simulink model "main"  (R2021a)
settings: Solver=ode113  StartTime=0.0  StopTime=6*3600  RelTol=1e-13  AbsTol=1e-14
values from neighbouring files (symbols this model uses):
  Const = createSimulinkBus(Const_1)    [initializeData.m]
  Earth = createSimulinkBus(Earth_1)    [initializeData.m]
  Sensors = createSimulinkBus(Sensors_1)    [initializeData.m]
  Spacecraft = createSimulinkBus(Spacecraft_1)    [initializeData.m]
undefined symbols (not defined in the file or in its folder): initCond
libraries: aerolibutil x25, vrlib x22, SADlibrary x22, dspsrcs4 x17, sharedtransform x8, simulink x6, pid_lib x3, simulink_extras x2, sharedTrackingLibrary x2, dspmathops x1, sharedutil x1
(part 1 of 2)
settings Model: SimulationMode=rapid-accelerator  Creator=matteo  LastModifiedBy=matteo
settings SolverCC: ZeroCrossControl=EnableAll  ZeroCrossAlgorithm=Adaptive  AlgebraicLoopSolver=TrustRegion  DecoupledContinuousIntegration=on
settings DebuggingCC: ReadBeforeWriteMsg=DisableAll  WriteAfterWriteMsg=DisableAll  WriteAfterReadMsg=DisableAll  MultiTaskDSMMsg=none  SFMachineParentedDataDiag=warning
settings ModelReferenceCC: UpdateModelReferenceTargets=IfOutOfDate
settings SFSimCC: SFSimEcho=off
settings SimscapeCC: SimscapeNormalizeSystem=off

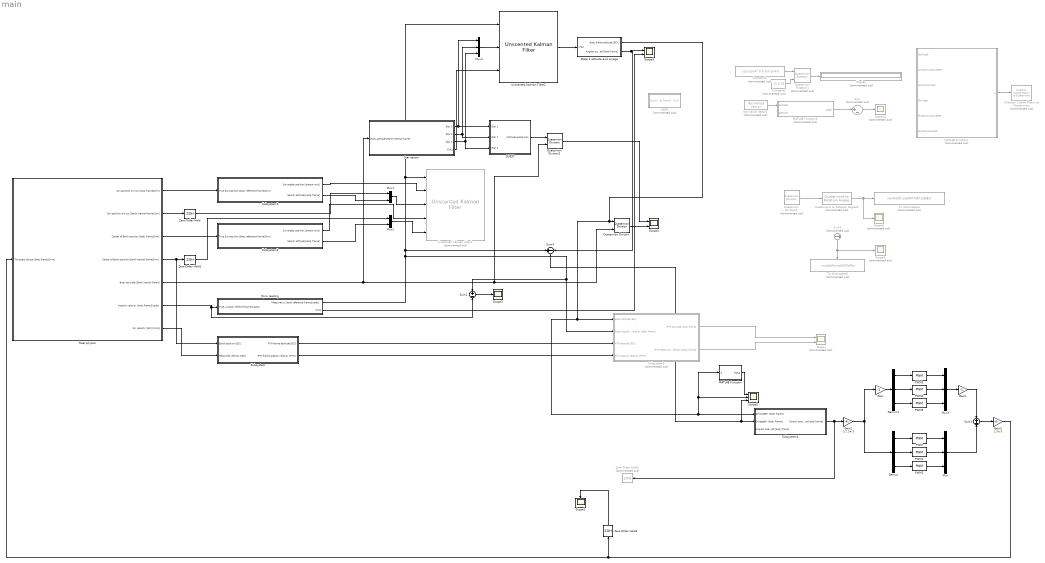
== system main ==
  Constant1 : Constant  Commented=on  Value=[1 0 0]
  Constant3 : Constant  Commented=on  Value=[cos(pi/4) 0 0 sin(pi/4)]
  Demux : Demux  Outputs=3
  Demux1 : Demux  Outputs=3
  Direction Cosine Matrix to Quaternions : sharedtransform/Direction Cosine Matrix  to Quaternions  Commented=on  aMode=0  action=None  tolerance=eps(2)
      settings: SourceProductBaseCode=AE,PW,DR,MT,UV,VE
  Display : Display  Commented=on
  Gain : Gain  Gain=-1
  Gain1 : Gain  Gain=-1
  Gain2 : Gain  Gain=1/2.5e-3
  Gain3 : Gain  Gain=2.5e-3
  Gyro reading : Subsystem
  MATLAB Function : MATLAB Function  TreatAsAtomicUnit=on
  MATLAB Function1 : MATLAB Function  Commented=on  TreatAsAtomicUnit=on
  MATLAB Function3 : MATLAB Function  Commented=on  TreatAsAtomicUnit=on
  MEKF : Subsystem  Commented=on
  Mux : Mux  Inputs=3
  Mux1 : Mux  Inputs=2
  Mux2 : Mux  Inputs=2
  Mux3 : Mux  Inputs=3
  Mux4 : Mux  Inputs=3
  Normalize Vector1 : vrlib/Utilities/Normalize Vector  Commented=on  maxzero=0
  PWM{,1..5} (6 alike) : simulink/Discontinuities/PWM  DisableCoverage=on  Period=.5  DisallowZeroDutyCycle=off  RunAtFixedTimeIntervals=on  SampleTime=.1
  QUEST : Subsystem
  Quaternion Division : aerolibutil/Quaternion Division
      settings: SourceProductBaseCode=AE
  Quaternion Division2 : aerolibutil/Quaternion Division
      settings: SourceProductBaseCode=AE
  Quaternion Division4 : aerolibutil/Quaternion Division  Commented=on
      settings: SourceProductBaseCode=AE
  Quaternion Rotation1 : aerolibutil/Quaternion Rotation  Commented=on
  Quaternions to Rotation Angles3 : sharedtransform/Quaternions to Rotation Angles  Commented=on  rotationOrder=ZYX  aMode=aMode
      settings: SourceProductBaseCode=AE,PW,DR,MT,UV,VE
  Real physics : Subsystem
  Scope : Scope  Commented=on  NumInputPorts=2
  Scope1 : Scope
  Scope10 : Scope  Commented=on
  Scope2 : Scope  NumInputPorts=3
  Scope3 : Scope
  Scope4 : Scope  NumInputPorts=2
  Scope5 : Scope  NumInputPorts=2
  Scope8 : Scope  Commented=on
  Scope9 : Scope  Commented=on
  Star sensor : Subsystem
  State 2 attitude and omega : Subsystem
  Subsystem : Subsystem
  Subsystem1 : Subsystem
  Subsystem2 : Subsystem  Commented=on
  Subsystem3 : Subsystem
  Subsystem4 : Subsystem
  Sum : Sum  Commented=on  Inputs=|+-
  Sum1 : Sum  Inputs=+-
  Sum2 : Sum  Commented=on  Inputs=-+
  Sum3 : Sum
  Sum4 : Sum  Inputs=+-
  To Workspace4 : ToWorkspace  Commented=on  VariableName=nonAdditiveUKFAttitudeErr  SaveFormat=Timeseries  SampleTime=-1
  To Workspace5 : ToWorkspace  Commented=on  VariableName=nonAdditiveUKFVelErr  SaveFormat=Timeseries  SampleTime=-1
  Unscented Kalman Filter1 : sharedTrackingLibrary/Unscented Kalman Filter  Commented=on  StateTransitionFcn=attitudePropagation  HasAdditiveProcessNoise=Nonadditive  ProcessNoise=(1e-1)^2*eye(6)  HasTimeVaryingProcessNoise=off  HasStateTransitionFcnExtraArgument=1  InitialState=[Spacecraft.initialAttitude' 0 0 0]'  InitialStateCovariance=1e-6*eye(7)  Alpha=1e-3  Beta=2  Kappa=0  MeasurementFcn1=simulateSunSensor  HasMeasurementEnablePort1=off  HasAdditiveMeasurementNoise1=Additive  MeasurementNoise1=(.1*pi/180)^2*eye(2)  HasTimeVaryingMeasurementNoise1=off  HasMeasurementFcnExtraArgument1=1  MeasurementFcn2=simulateEarthHorizonSensor  HasMeasurementEnablePort2=off  HasAdditiveMeasurementNoise2=Additive  MeasurementNoise2=(.1*pi/180)^2*eye(2)  HasTimeVaryingMeasurementNoise2=off  HasMeasurementFcnExtraArgument2=1  MeasurementFcn3=simulateSunSensor  HasMeasurementEnablePort3=off  HasAdditiveMeasurementNoise3=Additive  MeasurementNoise3=(.1*pi/180)^2*eye(2)  HasTimeVaryingMeasurementNoise3=off  HasMeasurementFcnExtraArgument3=1  MeasurementFcn4=myMeasurementFcn  HasMeasurementEnablePort4=off  HasAdditiveMeasurementNoise4=Additive  MeasurementNoise4=1  HasTimeVaryingMeasurementNoise4=off  HasMeasurementFcnExtraArgument4=0  MeasurementFcn5=myMeasurementFcn  HasMeasurementEnablePort5=off  HasAdditiveMeasurementNoise5=Additive  MeasurementNoise5=1  HasTimeVaryingMeasurementNoise5=off  HasMeasurementFcnExtraArgument5=0  EnableMultirate=on  StateTransitionFcnSampleTime=.01  MeasurementFcn1SampleTime=Sensors.sunSensorSamplingFreq  MeasurementFcn2SampleTime=Sensors.sunSensorSamplingFreq  MeasurementFcn3SampleTime=Sensors.sunSensorSamplingFreq  MeasurementFcn4SampleTime=1  MeasurementFcn5SampleTime=1  UseCurrentEstimator=on  OutputStateCovariance=off  DataType=double  SampleTime=0.01  NumberOfMeasurements=2
      settings: SourceProductBaseCode=CT,DR,TF,ID,LP,NV,AR,RO,RR,UV,VE
  Unscented Kalman Filter2 : sharedTrackingLibrary/Unscented Kalman Filter  StateTransitionFcn=attitudePropagation  HasAdditiveProcessNoise=Nonadditive  ProcessNoise=(1e-4)^2*eye(6)  HasTimeVaryingProcessNoise=off  HasStateTransitionFcnExtraArgument=1  InitialState=[Spacecraft.initialAttitude' 0 0 0]'  InitialStateCovariance=1e-6*eye(7)  Alpha=1e-3  Beta=2  Kappa=0  MeasurementFcn1=simulateStarSensor  HasMeasurementEnablePort1=off  HasAdditiveMeasurementNoise1=Additive  MeasurementNoise1=(.1*pi/180)^2*eye(6)  HasTimeVaryingMeasurementNoise1=off  HasMeasurementFcnExtraArgument1=1  MeasurementFcn2=simulateEarthHorizonSensor  HasMeasurementEnablePort2=off  HasAdditiveMeasurementNoise2=Additive  MeasurementNoise2=(.1*pi/180)^2*eye(2)  HasTimeVaryingMeasurementNoise2=off  HasMeasurementFcnExtraArgument2=1  MeasurementFcn3=simulateSunSensor  HasMeasurementEnablePort3=off  HasAdditiveMeasurementNoise3=Additive  MeasurementNoise3=(.1*pi/180)^2*eye(2)  HasTimeVaryingMeasurementNoise3=off  HasMeasurementFcnExtraArgument3=1  MeasurementFcn4=myMeasurementFcn  HasMeasurementEnablePort4=off  HasAdditiveMeasurementNoise4=Additive  MeasurementNoise4=1  HasTimeVaryingMeasurementNoise4=off  HasMeasurementFcnExtraArgument4=0  MeasurementFcn5=myMeasurementFcn  HasMeasurementEnablePort5=off  HasAdditiveMeasurementNoise5=Additive  MeasurementNoise5=1  HasTimeVaryingMeasurementNoise5=off  HasMeasurementFcnExtraArgument5=0  EnableMultirate=on  StateTransitionFcnSampleTime=.01  MeasurementFcn1SampleTime=1  MeasurementFcn2SampleTime=Sensors.sunSensorSamplingFreq  MeasurementFcn3SampleTime=Sensors.sunSensorSamplingFreq  MeasurementFcn4SampleTime=1  MeasurementFcn5SampleTime=1  UseCurrentEstimator=off  OutputStateCovariance=off  DataType=double  SampleTime=0.01  NumberOfMeasurements=1
      settings: SourceProductBaseCode=CT,DR,TF,ID,LP,NV,AR,RO,RR,UV,VE
  Zero-Order Hold : ZeroOrderHold  SampleTime=Sensors.sunSensorSamplingFreq
  Zero-Order Hold1 : ZeroOrderHold  SampleTime=Sensors.sunSensorSamplingFreq
  Zero-Order Hold2 : ZeroOrderHold  Commented=on  SampleTime=.01
  Zero-Order Hold3 : ZeroOrderHold  SampleTime=.01
  wires:
  Real physics/6(Angular velocity [body frame][rad/s]) -> Sum1/2, Gyro reading/1(True ω [body refrence frame][rad/s])
  Real physics/2(Sun position wrt s/c [Earth inertial frame][km]) -> Zero-Order Hold/1
  Real physics/4(Center of Earth position [Earth inertial frame][km]) -> Subsystem/1(Earth position [ECI]), Zero-Order Hold1/1
  Sum2/1 -> To Workspace5/1, Scope9/1
  Quaternions to Rotation Angles3/1 -> Scope8/1, To Workspace4/1
  Quaternion Division4/1 -> Quaternions to Rotation Angles3/1
  Real physics/3(Center of Earth position [body frame][km]) -> Subsystem3/1(True Sun position [body reference frame][km])
  Zero-Order Hold/1 -> Mux1/1
  Zero-Order Hold1/1 -> Mux2/1
  Normalize Vector1/1 -> MATLAB Function3/1(earthECI)
  MATLAB Function3/1(angle) -> Sum/1
  Sum/1 -> Scope10/1
  Real physics/7(S/c velocity [ECI][kim/s]) -> Subsystem/2(Measured velocity [ECI])
  Demux/1 -> PWM/1
  Demux/3 -> PWM2/1
  Demux/2 -> PWM1/1
  PWM/1 -> Mux/1
  PWM1/1 -> Mux/2
  PWM2/1 -> Mux/3
  Subsystem1/1(Sun angles position [sensor axis]) -> Unscented Kalman Filter1/2
  Real physics/1(Sun position wrt s/c [body frame][km]) -> Subsystem1/1(True Sun position [body reference frame][km])
  Subsystem3/2(Sensor attitude [body frame]) -> Mux2/2
  Subsystem3/1(Sun angles position [sensor axis]) -> Unscented Kalman Filter1/4
  Subsystem1/2(Sensor attitude [body frame]) -> Mux1/2
  Constant3/1 -> Quaternion Rotation1/1
  Constant1/1 -> Quaternion Rotation1/2
  Quaternion Rotation1/1 -> Display/1
  Mux1/1 -> Unscented Kalman Filter1/3
  Mux2/1 -> Unscented Kalman Filter1/5
  Sum3/1 -> Gain3/1
  State 2 attitude and omega/1(Body frame attitude [ECI]) -> MATLAB Function/1(q), Scope2/2, Subsystem4/1(AttitudeErr [body frame]), Subsystem2/1(Body attitude [ECI]), Quaternion Division/1
  Gyro reading/1(Measured ω [body reference frame][rad/s]) -> Sum4/1, Unscented Kalman Filter2/1, Unscented Kalman Filter1/1, Sum1/1, Subsystem2/2(Body angular velocity [body frame])
  Subsystem/1(RTH frame attitude [ECI]) -> Subsystem2/3(RTH attitude [ECI])
  Subsystem/2("RTH frame angular velocity [RTH] ") -> Subsystem2/4(RTH angular velocity [RTH])
  Subsystem2/1(RTH attitude [body frame]) -> Scope/1
  Subsystem2/2(RTH relative angular velocity [body frame]) -> Scope/2
  Sum1/1 -> Scope3/1
  PWM3/1 -> Mux3/1
  PWM5/1 -> Mux3/3
  Demux1/2 -> PWM4/1
  PWM4/1 -> Mux3/2
  Demux1/1 -> PWM3/1
  Demux1/3 -> PWM5/1
  Gain/1 -> Demux1/1
  Mux3/1 -> Gain1/1
  Gain1/1 -> Sum3/1
  Mux/1 -> Sum3/2
  Subsystem4/1(Control torque [body frame]) -> Zero-Order Hold2/1, Gain2/1
  Zero-Order Hold3/1 -> Scope1/1
  Gain2/1 -> Gain/1, Demux/1
  Gain3/1 -> Zero-Order Hold3/1, Real physics/1(Thrusters torque [body frame][N m])
  MATLAB Function/1(theta) -> Scope2/1
  MATLAB Function1/1(A) -> Direction Cosine Matrix to Quaternions/1
  Real physics/5(Body attitude [Earth inertial frame]) -> Quaternion Division2/2, Quaternion Division/2, Star sensor/1(Body attitude [Earth inertial frame])
  Quaternion Division/1 -> Scope4/2
  Star sensor/1(Star 1) -> Mux4/1, QUEST/1(Star 1)
  Star sensor/2(Star 2) -> QUEST/2(Star 2), Mux4/2
  Star sensor/3(Star 3) -> QUEST/3(Star 3), Mux4/3
  QUEST/1(Attitude quaternion) -> Quaternion Division2/1
  Quaternion Division2/1 -> Scope4/1
  Mux4/1 -> Unscented Kalman Filter2/2
  Star sensor/4(Out1) -> Unscented Kalman Filter2/3
  Unscented Kalman Filter2/1 -> State 2 attitude and omega/1(xHat)
  Gyro reading/2(Out1) -> Scope5/2
  State 2 attitude and omega/2(Angolar speed [body frame]) -> Sum4/2, Scope5/1
  Sum4/1 -> Subsystem4/2(OmegaErr [body frame]), Scope2/3

== system main/Gyro reading ==
  True ω [body refrence frame][rad/s] : Inport
  Cumulative Sum : dspmathops/Cumulative Sum  dim=Channels (running sum)  reset_popup=None  roundingMode=Floor  overflowMode=off  outputDataTypeStr=Inherit: Same as accumulator  outputMin=[]  outputMax=[]  outputLastDataTypeStr=Inherit: Same as accumulator
  Gain : Gain  Gain=sqrt(0.01)
  Random Source : dspsrcs4/Random Source  SrcType=Gaussian  NormMethod=Ziggurat  CltLength=12  MinVal=0  MaxVal=1  MeanVal=0  VarVal=(1e-4)^2  RepMode=Not repeatable  rawSeed=1  IsInherit=off  SampMode=Discrete  SampTime=0.01  SampFrame=3  DataType=Double  OutComplex=Real  OutputFrames=off
  Random Source1 : dspsrcs4/Random Source  SrcType=Gaussian  NormMethod=Ziggurat  CltLength=12  MinVal=0  MaxVal=1  MeanVal=0  VarVal=(1e-4)^2  RepMode=Not repeatable  rawSeed=1  IsInherit=off  SampMode=Discrete  SampTime=0.01  SampFrame=3  DataType=Double  OutComplex=Real  OutputFrames=off
  Sum : Sum  Inputs=+++
  Zero-Order Hold : ZeroOrderHold  SampleTime=.01
  Measured ω [body reference frame][rad/s] : Outport
  Out1 : Outport  Port=2
  wires:
  Sum/1 -> Measured ω [body reference frame][rad/s]/1
  True ω [body refrence frame][rad/s]/1 -> Zero-Order Hold/1
  Zero-Order Hold/1 -> Sum/2
  Cumulative Sum/1 -> Out1/1, Sum/1
  Gain/1 -> Cumulative Sum/1
  Random Source/1 -> Sum/3
  Random Source1/1 -> Gain/1

== system main/MEKF ==
  note: With
      | $G(t)= \left[ \begin{array}{cccccc} -1 \\ & -1 \\ & & -1 \\ & & & 1 \\ & & & & 1 \\ & & & & & 1 \end{array} \right] \quad \text{and} \quad Q(t) = \left[ \begin{array}{cccccc} \sigma_v^2 \\ & \sigma_v^2 \\ & & \sigma_v^2 \\ & & & \sigma_u^2 \\ & & & & \sigma_u^2 \\ & & & & & \sigma_u^2 \end{array} \right]$
  Gyro [rad/s] [body frame] : Inport
  G*Q*G' : Constant  Value="diag([1  1  1  1  1  1 ])"
  Gain : Gain  Gain=0.5
  Integrator : Integrator  InitialConditionSource=external
  Integrator1 : Integrator  InitialConditionSource=external
  MATLAB Function : MATLAB Function  TreatAsAtomicUnit=on
  MATLAB Function1 : MATLAB Function  TreatAsAtomicUnit=on
  MATLAB Function2 : MATLAB Function  TreatAsAtomicUnit=on
  Product : Product
  Product1 : Product
  Product2 : Product
  Sum : Sum  Inputs=+++
  Transpose : Math  Operator=transpose  SaturateOnIntegerOverflow=on
  Out1 : Outport
  wires:
  Gyro [rad/s] [body frame]/1 -> MATLAB Function1/1(v), Out1/1, Product/2
  MATLAB Function/1(Q) -> Product/1
  Product/1 -> Gain/1
  Gain/1 -> Integrator/1
  Integrator/1 -> MATLAB Function/1(q)
  MATLAB Function1/1(vCross) -> MATLAB Function2/1(omegaCross)
  MATLAB Function2/1(F) -> Product1/1, Transpose/1
  Integrator1/1 -> Product1/2, Product2/1
  Transpose/1 -> Product2/2
  Product1/1 -> Sum/2
  Product2/1 -> Sum/3
  Sum/1 -> Integrator1/1
  G*Q*G'/1 -> Sum/1

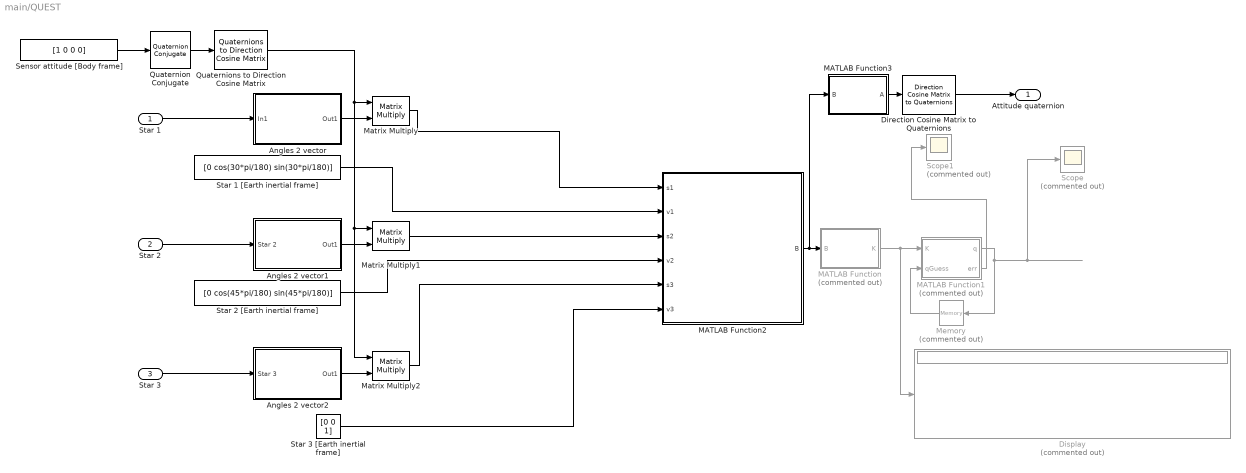
== system main/QUEST ==
  Star 1 : Inport
  Star 2 : Inport  Port=2
  Star 3 : Inport  Port=3
  Angles 2 vector : Subsystem
  Angles 2 vector1 : Subsystem
  Angles 2 vector2 : Subsystem
  Direction Cosine Matrix to Quaternions : sharedtransform/Direction Cosine Matrix  to Quaternions  aMode=0  action=None  tolerance=eps(2)
      settings: SourceProductBaseCode=AE,PW,DR,MT,UV,VE
  Display : Display  Commented=on
  MATLAB Function : MATLAB Function  Commented=on  TreatAsAtomicUnit=on
  MATLAB Function1 : MATLAB Function  Commented=on  TreatAsAtomicUnit=on
  MATLAB Function2 : MATLAB Function  TreatAsAtomicUnit=on
  MATLAB Function3 : MATLAB Function  TreatAsAtomicUnit=on
  Matrix Multiply : Product  Multiplication=Matrix(*)
  Matrix Multiply1 : Product  Multiplication=Matrix(*)
  Matrix Multiply2 : Product  Multiplication=Matrix(*)
  Memory : Memory  Commented=on  InitialCondition=[1 0 0 0]
  Quaternion Conjugate : aerolibutil/Quaternion Conjugate
      settings: SourceProductBaseCode=AE
  Quaternions to Direction Cosine Matrix : sharedtransform/Quaternions to  Direction Cosine Matrix  aMode=aMode
      settings: SourceProductBaseCode=AE,PW,DR,MT,UV,VE
  Scope : Scope  Commented=on
  Scope1 : Scope  Commented=on
  Sensor attitude [Body frame] : Constant  Value=[1 0 0 0]
  Star 1 [Earth inertial frame] : Constant  Value=[0 cos(30*pi/180) sin(30*pi/180)]
  Star 2 [Earth inertial frame] : Constant  Value=[0 cos(45*pi/180) sin(45*pi/180)]
  Star 3 [Earth inertial frame] : Constant  Value=[0 0 1]
  Attitude quaternion : Outport
  wires:
  Star 1/1 -> Angles 2 vector/1(In1)
  Star 2/1 -> Angles 2 vector1/1(Star 2)
  Star 3/1 -> Angles 2 vector2/1(Star 3)
  Star 1 [Earth inertial frame]/1 -> MATLAB Function2/2(v1)
  Angles 2 vector/1(Out1) -> Matrix Multiply/2
  Star 2 [Earth inertial frame]/1 -> MATLAB Function2/4(v2)
  Star 3 [Earth inertial frame]/1 -> MATLAB Function2/6(v3)
  MATLAB Function2/1(B) -> MATLAB Function3/1(B), MATLAB Function/1(B)
  MATLAB Function/1(K) -> Display/1, MATLAB Function1/1(K)
  MATLAB Function1/1(q) -> Memory/1, Scope/1
  Sensor attitude [Body frame]/1 -> Quaternion Conjugate/1
  Quaternion Conjugate/1 -> Quaternions to Direction Cosine Matrix/1
  Quaternions to Direction Cosine Matrix/1 -> Matrix Multiply2/1, Matrix Multiply1/1, Matrix Multiply/1
  Matrix Multiply/1 -> MATLAB Function2/1(s1)
  Angles 2 vector2/1(Out1) -> Matrix Multiply2/2
  Matrix Multiply2/1 -> MATLAB Function2/5(s3)
  Matrix Multiply1/1 -> MATLAB Function2/3(s2)
  Angles 2 vector1/1(Out1) -> Matrix Multiply1/2
  Memory/1 -> MATLAB Function1/2(qGuess)
  MATLAB Function1/2(err) -> Scope1/1
  MATLAB Function3/1(A) -> Direction Cosine Matrix to Quaternions/1
  Direction Cosine Matrix to Quaternions/1 -> Attitude quaternion/1

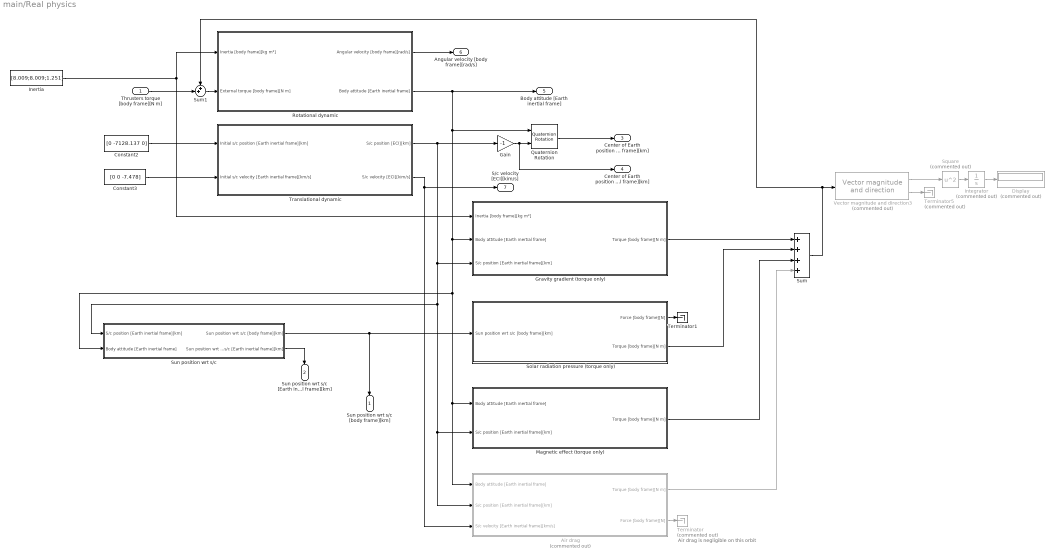
== system main/Real physics ==
  note: Air drag is negligible on this orbit
  Thrusters torque [body frame][N m] : Inport  Unit=N*m
  Air drag : Subsystem  Commented=on
  Constant2 : Constant  Value=[0 -7128.137 0]
  Constant3 : Constant  Value=[0 0 -7.478]
  Display : Display  Commented=on
  Gain : Gain  Gain=-1
  Gravity gradient (torque only) : Subsystem
      settings: PortSchema="{\"entries\":[{\"content\":{\"sides\":[{\"content\":{\"connectorIds\":[\"Out1\"]},\"type\":\"ConnectorPlacement.EquallySpacedRectSide\",\"uuid\":\"f1f9fb06-69b8-4265-b1e3-1bc99765f445\"},{\"content\":{\"connectorIds\":[\"In1\",\"In2\",\"In3\"],\"side\":\"RIGHT\"},\"type\":\"ConnectorPlacement.EquallySpacedRectSide\",\"uuid\":\"95872401-8fe8-493a-a743-72ee2e043305\"},{\"content\":{\"connectorIds\":[],\"side\":\"TOP\"},\"type\":\"ConnectorPlacement.EquallySpacedRectSide\",\"uuid\":\"a2f933f3-d116-4556-b216-8e543aff18f5\"},{\"content\":{\"connectorIds\":[],\"side\":\"HIDDEN\"},\"type\":\"ConnectorPlacement.EquallySpacedRectSide\",\"uuid\":\"93d45030-e624-494e-a335-b0ea445a7c18\"}]},\"type\":\"ConnectorPlacement.EquallySpacedConnector\",\"uuid\":\"bbb7bc93-29be-48e8-9ed7-f6b41cc2b7e1\"}],\"packageUris\":[\"http://schema.mathworks.com/mf0/Connector/R2020b\"],\"version\":\"1.0\"}"
  Inertia : Constant  Value=[8.009;8.009;1.251]
  Integrator : Integrator  Commented=on
  Magnetic effect (torque only) : Subsystem
  Quaternion Rotation : aerolibutil/Quaternion Rotation
  Rotational dynamic : Subsystem
  Solar radiation pressure (torque only) : Subsystem
  Square : Math  Commented=on  Operator=square  SaturateOnIntegerOverflow=on
  Sum : Sum  Inputs=++++
  Sum1 : Sum  Inputs=++|
  Sun position wrt s/c : Subsystem
  Terminator : Terminator  Commented=on
  Terminator1 : Terminator
  Terminator5 : Terminator  Commented=on
  Translational dynamic : Subsystem
  Vector magnitude and direction3 : SADlibrary/Vector magnitude and direction  Commented=on  SystemSampleTime=-1  VariantActivationTime=update diagram  Latency=0  AutoFrameSizeCalculation=off
  Sun position wrt s/c [body frame][km] : Outport  OutDataTypeStr=double  Unit=km
  Sun position wrt s/c [Earth inertial frame][km] : Outport  Port=2
  Center of Earth position [body frame][km] : Outport  Port=3
  Center of Earth position [Earth inertial frame][km] : Outport  Port=4
  Body attitude [Earth inertial frame] : Outport  Port=5
  Angular velocity [body frame][rad/s] : Outport  Port=6
  S/c velocity [ECI][kim/s] : Outport  Port=7
  wires:
  Inertia/1 -> Gravity gradient (torque only)/1(Inertia [body frame][kg m²]), Rotational dynamic/1(Inertia [body frame][kg m²])
  Rotational dynamic/1(Angular velocity [body frame][rad/s]) -> Angular velocity [body frame][rad/s]/1
  Constant2/1 -> Translational dynamic/1(Initial s/c position [Earth inertial frame][km])
  Constant3/1 -> Translational dynamic/2(Initial s/c velocity [Earth inertial frame][km/s])
  Rotational dynamic/2(Body attitude [Earth inertial frame]) -> Body attitude [Earth inertial frame]/1, Quaternion Rotation/1, Air drag/1(Body attitude [Earth inertial frame]), Magnetic effect (torque only)/1(Body attitude [Earth inertial frame]), Sun position wrt s/c/2(Body attitude [Earth inertial frame]), Gravity gradient (torque only)/2(Body attitude [Earth inertial frame])
  Translational dynamic/1(S/c position [ECI][km]) -> Gain/1, Gravity gradient (torque only)/3(S/c position [Earth inertial frame][km]), Sun position wrt s/c/1(S/c position [Earth inertial frame][km]), Air drag/2(S/c position [Earth inertial frame][km]), Magnetic effect (torque only)/2(S/c position [Earth inertial frame][km])
  Sum/1 -> Sum1/1, Vector magnitude and direction3/1
  Air drag/2(Force [body frame][N]) -> Terminator/1
  Solar radiation pressure (torque only)/1(Force [body frame][N]) -> Terminator1/1
  Sun position wrt s/c/1(Sun position wrt s/c [body frame][km]) -> Solar radiation pressure (torque only)/1(Sun position wrt s/c [body frame][km]), Sun position wrt s/c [body frame][km]/1
  Solar radiation pressure (torque only)/2(Torque [body frame][N m]) -> Sum/2
  Magnetic effect (torque only)/1(Torque [body frame][N m]) -> Sum/3
  Air drag/1(Torque [body frame][N m]) -> Sum/4
  Gravity gradient (torque only)/1(Torque [body frame][N m]) -> Sum/1
  Gain/1 -> Center of Earth position [Earth inertial frame][km]/1, Quaternion Rotation/2
  Quaternion Rotation/1 -> Center of Earth position [body frame][km]/1
  Sun position wrt s/c/2(Sun position wrt s/c [Earth inertial frame][km]) -> Sun position wrt s/c [Earth inertial frame][km]/1
  Thrusters torque [body frame][N m]/1 -> Sum1/2
  Sum1/1 -> Rotational dynamic/2(External torque [body frame][N m])
  Vector magnitude and direction3/1 -> Square/1
  Vector magnitude and direction3/2 -> Terminator5/1
  Square/1 -> Integrator/1
  Integrator/1 -> Display/1
  Translational dynamic/2(S/c velocity [ECI][kim/s]) -> S/c velocity [ECI][kim/s]/1, Air drag/3(S/c velocity [Earth inertial frame][km/s])

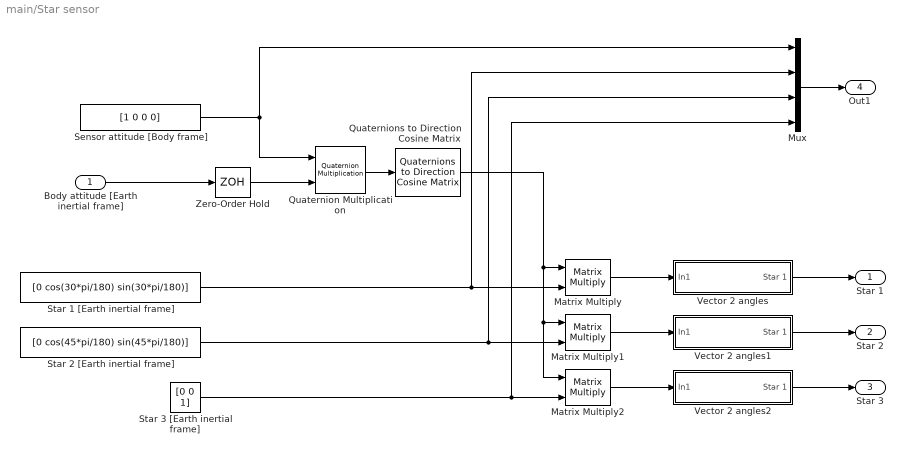
== system main/Star sensor ==
  Body attitude [Earth inertial frame] : Inport
  Matrix Multiply : Product  Multiplication=Matrix(*)
  Matrix Multiply1 : Product  Multiplication=Matrix(*)
  Matrix Multiply2 : Product  Multiplication=Matrix(*)
  Mux : Mux
  Quaternion Multiplication : aerolibutil/Quaternion Multiplication
  Quaternions to Direction Cosine Matrix : sharedtransform/Quaternions to  Direction Cosine Matrix  aMode=aMode
      settings: SourceProductBaseCode=AE,PW,DR,MT,UV,VE
  Sensor attitude [Body frame] : Constant  Value=[1 0 0 0]
  Star 1 [Earth inertial frame] : Constant  Value=[0 cos(30*pi/180) sin(30*pi/180)]
  Star 2 [Earth inertial frame] : Constant  Value=[0 cos(45*pi/180) sin(45*pi/180)]
  Star 3 [Earth inertial frame] : Constant  Value=[0 0 1]
  Vector 2 angles : Subsystem
  Vector 2 angles1 : Subsystem
  Vector 2 angles2 : Subsystem
  Zero-Order Hold : ZeroOrderHold
  Star 1 : Outport
  Star 2 : Outport  Port=2
  Star 3 : Outport  Port=3
  Out1 : Outport  Port=4
  wires:
  Body attitude [Earth inertial frame]/1 -> Zero-Order Hold/1
  Sensor attitude [Body frame]/1 -> Mux/1, Quaternion Multiplication/1
  Quaternion Multiplication/1 -> Quaternions to Direction Cosine Matrix/1
  Star 1 [Earth inertial frame]/1 -> Matrix Multiply/2, Mux/2
  Star 2 [Earth inertial frame]/1 -> Mux/3, Matrix Multiply1/2
  Star 3 [Earth inertial frame]/1 -> Mux/4, Matrix Multiply2/2
  Quaternions to Direction Cosine Matrix/1 -> Matrix Multiply2/1, Matrix Multiply1/1, Matrix Multiply/1
  Matrix Multiply/1 -> Vector 2 angles/1(In1)
  Matrix Multiply2/1 -> Vector 2 angles2/1(In1)
  Matrix Multiply1/1 -> Vector 2 angles1/1(In1)
  Vector 2 angles1/1(Star 1) -> Star 2/1
  Vector 2 angles2/1(Star 1) -> Star 3/1
  Vector 2 angles/1(Star 1) -> Star 1/1
  Mux/1 -> Out1/1
  Zero-Order Hold/1 -> Quaternion Multiplication/2

== system main/State 2 attitude and omega ==
  xHat : Inport
  Demux1 : Demux  Outputs=7
  Mux2 : Mux
  Mux3 : Mux  Inputs=3
  Body frame attitude [ECI] : Outport
  Angolar speed [body frame] : Outport  Port=2
  wires:
  Mux2/1 -> Body frame attitude [ECI]/1
  Demux1/2 -> Mux2/2
  Mux3/1 -> Angolar speed [body frame]/1
  Demux1/7 -> Mux3/3
  Demux1/1 -> Mux2/1
  Demux1/3 -> Mux2/3
  Demux1/5 -> Mux3/1
  xHat/1 -> Demux1/1
  Demux1/6 -> Mux3/2
  Demux1/4 -> Mux2/4

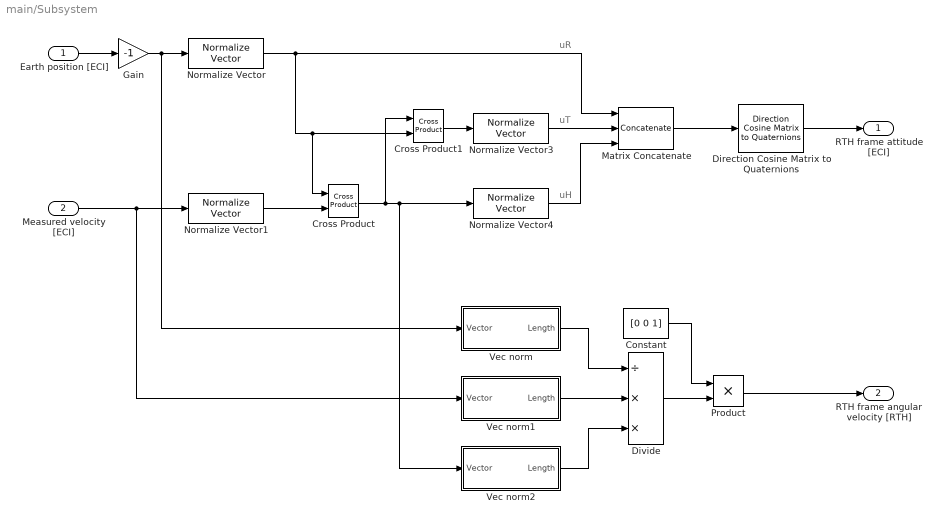
== system main/Subsystem ==
  note: uR
  note: uT
  note: uH
  Earth position [ECI] : Inport
  Measured velocity [ECI] : Inport  Port=2
  Constant : Constant  Value=[0 0 1]
  Cross Product : vrlib/Utilities/Cross Product
  Cross Product1 : vrlib/Utilities/Cross Product
  Direction Cosine Matrix to Quaternions : sharedtransform/Direction Cosine Matrix  to Quaternions  aMode=0  action=None  tolerance=eps(2)
      settings: SourceProductBaseCode=AE,PW,DR,MT,UV,VE
  Divide : Product  Inputs=/**
  Gain : Gain  Gain=-1
  Matrix Concatenate : Concatenate  NumInputs=3  Mode=Multidimensional array  ConcatenateDimension=2
  Normalize Vector{,1,3..4} (4 alike) : vrlib/Utilities/Normalize Vector  maxzero=0
  Product : Product
  Vec norm : Subsystem
  Vec norm1 : Subsystem
  Vec norm2 : Subsystem
  RTH frame attitude [ECI] : Outport
  "RTH frame angular velocity [RTH] " : Outport  Port=2
  wires:
  Matrix Concatenate/1 -> Direction Cosine Matrix to Quaternions/1
  Direction Cosine Matrix to Quaternions/1 -> RTH frame attitude [ECI]/1
  Earth position [ECI]/1 -> Gain/1
  Cross Product/1 -> Vec norm2/1(Vector), Normalize Vector4/1, Cross Product1/1
  Normalize Vector/1 -> Matrix Concatenate/1, Cross Product/1, Cross Product1/2
  Normalize Vector4/1 -> Matrix Concatenate/3
  Normalize Vector3/1 -> Matrix Concatenate/2
  Measured velocity [ECI]/1 -> Vec norm1/1(Vector), Normalize Vector1/1
  Cross Product1/1 -> Normalize Vector3/1
  Vec norm/1(Length) -> Divide/1
  Vec norm1/1(Length) -> Divide/2
  Vec norm2/1(Length) -> Divide/3
  Divide/1 -> Product/2
  Product/1 -> "RTH frame angular velocity [RTH] "/1
  Normalize Vector1/1 -> Cross Product/2
  Gain/1 -> Normalize Vector/1, Vec norm/1(Vector)
  Constant/1 -> Product/1

== system main/Subsystem1 ==
  True Sun position [body reference frame][km] : Inport
  MATLAB Function1 : MATLAB Function  TreatAsAtomicUnit=on
  Sun sensor reading1 : Subsystem
  Sun sensor reading2 : Subsystem
  Sun sensor reading3 : Subsystem
  Sun sensor reading4 : Subsystem
  Sun sensor reading5 : Subsystem
  Sun sensor reading6 : Subsystem
  Sun angles position [sensor axis] : Outport  PortDimensions=2
  Sensor attitude [body frame] : Outport  Port=2  PortDimensions=4
  wires:
  True Sun position [body reference frame][km]/1 -> Sun sensor reading3/1(True Sun position [body reference frame][km]), Sun sensor reading1/1(True Sun position [body reference frame][km]), Sun sensor reading2/1(True Sun position [body reference frame][km]), Sun sensor reading6/1(True Sun position [body reference frame][km]), Sun sensor reading5/1(True Sun position [body reference frame][km]), Sun sensor reading4/1(True Sun position [body reference frame][km])
  MATLAB Function1/2(sensAtt) -> Sensor attitude [body frame]/1
  Sun sensor reading2/1(Sun angles position [sensor axis]) -> MATLAB Function1/2(s2)
  Sun sensor reading1/1(Sun angles position [sensor axis]) -> MATLAB Function1/1(s1)
  Sun sensor reading3/1(Sun angles position [sensor axis]) -> MATLAB Function1/3(s3)
  Sun sensor reading4/1(Sun angles position [sensor axis]) -> MATLAB Function1/4(s4)
  Sun sensor reading5/1(Sun angles position [sensor axis]) -> MATLAB Function1/5(s5)
  Sun sensor reading6/1(Sun angles position [sensor axis]) -> MATLAB Function1/6(s6)
  MATLAB Function1/1(s) -> Sun angles position [sensor axis]/1

== system main/Subsystem2 ==
  Body attitude [ECI] : Inport
  Body angular velocity [body frame] : Inport  Port=2
  RTH attitude [ECI] : Inport  Port=3
  RTH angular velocity [RTH] : Inport  Port=4
  Quaternion Conjugate : aerolibutil/Quaternion Conjugate
      settings: SourceProductBaseCode=AE
  Quaternion Multiplication : aerolibutil/Quaternion Multiplication
  Quaternion Rotation : aerolibutil/Quaternion Rotation
  Sum1 : Sum  Inputs=+-
  RTH attitude [body frame] : Outport
  RTH relative angular velocity [body frame] : Outport  Port=2
  wires:
  Sum1/1 -> RTH relative angular velocity [body frame]/1
  Body angular velocity [body frame]/1 -> Sum1/2
  RTH attitude [ECI]/1 -> Quaternion Multiplication/1
  RTH angular velocity [RTH]/1 -> Quaternion Rotation/2
  Body attitude [ECI]/1 -> Quaternion Conjugate/1
  Quaternion Rotation/1 -> Sum1/1
  Quaternion Multiplication/1 -> Quaternion Rotation/1, RTH attitude [body frame]/1
  Quaternion Conjugate/1 -> Quaternion Multiplication/2

== system main/Subsystem3 ==
  True Sun position [body reference frame][km] : Inport
  MATLAB Function1 : MATLAB Function  TreatAsAtomicUnit=on
  Sun sensor reading1 : Subsystem
  Sun sensor reading2 : Subsystem
  Sun sensor reading3 : Subsystem
  Sun sensor reading4 : Subsystem
  Sun sensor reading5 : Subsystem
  Sun sensor reading6 : Subsystem
  Sun angles position [sensor axis] : Outport  PortDimensions=2
  Sensor attitude [body frame] : Outport  Port=2  PortDimensions=4
  wires:
  True Sun position [body reference frame][km]/1 -> Sun sensor reading3/1(True Sun position [body reference frame][km]), Sun sensor reading1/1(True Sun position [body reference frame][km]), Sun sensor reading2/1(True Sun position [body reference frame][km]), Sun sensor reading6/1(True Sun position [body reference frame][km]), Sun sensor reading5/1(True Sun position [body reference frame][km]), Sun sensor reading4/1(True Sun position [body reference frame][km])
  MATLAB Function1/2(sensAtt) -> Sensor attitude [body frame]/1
  Sun sensor reading2/1(Sun angles position [sensor axis]) -> MATLAB Function1/2(s2)
  Sun sensor reading1/1(Sun angles position [sensor axis]) -> MATLAB Function1/1(s1)
  Sun sensor reading3/1(Sun angles position [sensor axis]) -> MATLAB Function1/3(s3)
  Sun sensor reading4/1(Sun angles position [sensor axis]) -> MATLAB Function1/4(s4)
  Sun sensor reading5/1(Sun angles position [sensor axis]) -> MATLAB Function1/5(s5)
  Sun sensor reading6/1(Sun angles position [sensor axis]) -> MATLAB Function1/6(s6)
  MATLAB Function1/1(s) -> Sun angles position [sensor axis]/1

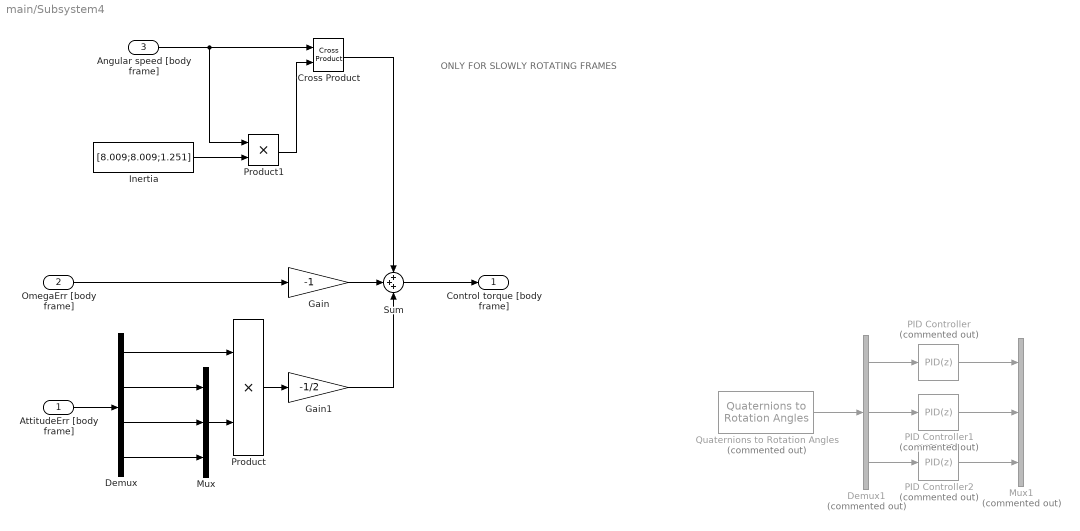
== system main/Subsystem4 ==
  note: ONLY FOR SLOWLY ROTATING FRAMES
  AttitudeErr [body frame] : Inport
  OmegaErr [body frame] : Inport  Port=2
  Angular speed [body frame] : Inport  Port=3
  Cross Product : vrlib/Utilities/Cross Product
  Demux : Demux
  Demux1 : Demux  Commented=on  Outputs=3
  Gain : Gain  Gain=-1
  Gain1 : Gain  Gain=-1/2
  Inertia : Constant  Value=[8.009;8.009;1.251]
  Mux : Mux  Inputs=3
  Mux1 : Mux  Commented=on  Inputs=3
  PID Controller : pid_lib/PID Controller  Commented=on  Controller=PID  Form=Parallel  TimeDomain=Discrete-time  UseExternalTs=off  SampleTime=-1  IntegratorMethod=Forward Euler  FilterMethod=Forward Euler  ControllerParametersSource=internal  P=1  I=1  D=0  UseFilter=on  N=100  TunerSelectOption=Transfer Function Based (PID Tuner App)  InitialConditionSource=internal  InitialConditionForIntegrator=0  InitialConditionForFilter=0  DifferentiatorICPrevScaledInput=0  ExternalReset=none  TrackingMode=off  Kt=1  LimitOutput=off  SatLimitsSource=internal  UpperSaturationLimit=inf  LowerSaturationLimit=-inf  LinearizeAsGain=on  AntiWindupMode=none  Kb=1  POutMin=[]  POutMax=[]  IOutMin=[]  IOutMax=[]  DOutMin=[]  DOutMax=[]  NOutMin=[]  NOutMax=[]  SumOutMin=[]  SumOutMax=[]  SaturationOutMin=[]  SaturationOutMax=[]  PParamMin=[]  PParamMax=[]  IParamMin=[]  IParamMax=[]  DParamMin=[]  DParamMax=[]  NParamMin=[]  NParamMax=[]  KbParamMin=[]  KbParamMax=[]  KtParamMin=[]  KtParamMax=[]  KbOutMin=[]  KbOutMax=[]  KtOutMin=[]  KtOutMax=[]  IntegratorOutMin=[]  IntegratorOutMax=[]  FilterOutMin=[]  FilterOutMax=[]  SumI1OutMin=[]  SumI1OutMax=[]  SumI2OutMin=[]  SumI2OutMax=[]  SumI3OutMin=[]  SumI3OutMax=[]  SumI4OutMin=[]  SumI4OutMax=[]  SumDOutMin=[]  SumDOutMax=[]  DifferentiatorOutMin=[]  DifferentiatorOutMax=[]  FilterDiffOutCoefMin=[]  FilterDiffOutCoefMax=[]  ReciprocalOutMin=[]  ReciprocalOutMax=[]  SumDenOutMin=[]  SumDenOutMax=[]  SumNumOutMin=[]  SumNumOutMax=[]  DivideOutMin=[]  DivideOutMax=[]  UdiffTsProdOutMin=[]  UdiffTsProdOutMax=[]  NTsProdOutMin=[]  NTsProdOutMax=[]  UintegralTsProdOutMin=[]  UintegralTsProdOutMax=[]  UngainTsProdOutMin=[]  UngainTsProdOutMax=[]  IntegratorContinuousStateAttributes=''  IntegratorStateMustResolveToSignalObject=off  IntegratorRTWStateStorageClass=Auto  FilterContinuousStateAttributes=''  FilterStateMustResolveToSignalObject=off  FilterRTWStateStorageClass=Auto  ParallelPVariant=InternalParameters  IdealPVariant=Disabled  IVariant=InternalParameters  DVariant=InternalParameters  IntegratorVariant=Discrete  SatVariant=Disabled  AWVariant=Passthrough  PCopyVariant=Disabled  TRVariant=Disabled  FdbkBlocksVariant=Forward  IdealPFdbkVariant=Disabled  SatFdbkVariant=Disabled  DerivativeFilterVariant=ForwardEulerFilter  NVariant=InternalParameters  NCopyVariant=Disabled  FilterICVariant=InternalICsFilter  IntegratorICVariant=InternalICs  ExternalResetVariant=Disabled  TRSumVariant=Passthrough  SumFdbkVariant=Disabled  SumVariant=Sum_PID  TsampFilterVariant=InternalTs  TsampNgainVariant=Passthrough  TsampIntegralVariant=Passthrough  ExternalSaturationOutDataTypeStr=Inherit: Same as second input
  PID Controller1 : pid_lib/PID Controller  Commented=on  Controller=PID  Form=Parallel  TimeDomain=Discrete-time  UseExternalTs=off  SampleTime=-1  IntegratorMethod=Forward Euler  FilterMethod=Forward Euler  ControllerParametersSource=internal  P=1  I=1  D=0  UseFilter=on  N=100  TunerSelectOption=Transfer Function Based (PID Tuner App)  InitialConditionSource=internal  InitialConditionForIntegrator=0  InitialConditionForFilter=0  DifferentiatorICPrevScaledInput=0  ExternalReset=none  TrackingMode=off  Kt=1  LimitOutput=off  SatLimitsSource=internal  UpperSaturationLimit=inf  LowerSaturationLimit=-inf  LinearizeAsGain=on  AntiWindupMode=none  Kb=1  POutMin=[]  POutMax=[]  IOutMin=[]  IOutMax=[]  DOutMin=[]  DOutMax=[]  NOutMin=[]  NOutMax=[]  SumOutMin=[]  SumOutMax=[]  SaturationOutMin=[]  SaturationOutMax=[]  PParamMin=[]  PParamMax=[]  IParamMin=[]  IParamMax=[]  DParamMin=[]  DParamMax=[]  NParamMin=[]  NParamMax=[]  KbParamMin=[]  KbParamMax=[]  KtParamMin=[]  KtParamMax=[]  KbOutMin=[]  KbOutMax=[]  KtOutMin=[]  KtOutMax=[]  IntegratorOutMin=[]  IntegratorOutMax=[]  FilterOutMin=[]  FilterOutMax=[]  SumI1OutMin=[]  SumI1OutMax=[]  SumI2OutMin=[]  SumI2OutMax=[]  SumI3OutMin=[]  SumI3OutMax=[]  SumI4OutMin=[]  SumI4OutMax=[]  SumDOutMin=[]  SumDOutMax=[]  DifferentiatorOutMin=[]  DifferentiatorOutMax=[]  FilterDiffOutCoefMin=[]  FilterDiffOutCoefMax=[]  ReciprocalOutMin=[]  ReciprocalOutMax=[]  SumDenOutMin=[]  SumDenOutMax=[]  SumNumOutMin=[]  SumNumOutMax=[]  DivideOutMin=[]  DivideOutMax=[]  UdiffTsProdOutMin=[]  UdiffTsProdOutMax=[]  NTsProdOutMin=[]  NTsProdOutMax=[]  UintegralTsProdOutMin=[]  UintegralTsProdOutMax=[]  UngainTsProdOutMin=[]  UngainTsProdOutMax=[]  IntegratorContinuousStateAttributes=''  IntegratorStateMustResolveToSignalObject=off  IntegratorRTWStateStorageClass=Auto  FilterContinuousStateAttributes=''  FilterStateMustResolveToSignalObject=off  FilterRTWStateStorageClass=Auto  ParallelPVariant=InternalParameters  IdealPVariant=Disabled  IVariant=InternalParameters  DVariant=InternalParameters  IntegratorVariant=Discrete  SatVariant=Disabled  AWVariant=Passthrough  PCopyVariant=Disabled  TRVariant=Disabled  FdbkBlocksVariant=Forward  IdealPFdbkVariant=Disabled  SatFdbkVariant=Disabled  DerivativeFilterVariant=ForwardEulerFilter  NVariant=InternalParameters  NCopyVariant=Disabled  FilterICVariant=InternalICsFilter  IntegratorICVariant=InternalICs  ExternalResetVariant=Disabled  TRSumVariant=Passthrough  SumFdbkVariant=Disabled  SumVariant=Sum_PID  TsampFilterVariant=InternalTs  TsampNgainVariant=Passthrough  TsampIntegralVariant=Passthrough  ExternalSaturationOutDataTypeStr=Inherit: Same as second input
  PID Controller2 : pid_lib/PID Controller  Commented=on  Controller=PID  Form=Parallel  TimeDomain=Discrete-time  UseExternalTs=off  SampleTime=-1  IntegratorMethod=Forward Euler  FilterMethod=Forward Euler  ControllerParametersSource=internal  P=1  I=1  D=0  UseFilter=on  N=100  TunerSelectOption=Transfer Function Based (PID Tuner App)  InitialConditionSource=internal  InitialConditionForIntegrator=0  InitialConditionForFilter=0  DifferentiatorICPrevScaledInput=0  ExternalReset=none  TrackingMode=off  Kt=1  LimitOutput=off  SatLimitsSource=internal  UpperSaturationLimit=inf  LowerSaturationLimit=-inf  LinearizeAsGain=on  AntiWindupMode=none  Kb=1  POutMin=[]  POutMax=[]  IOutMin=[]  IOutMax=[]  DOutMin=[]  DOutMax=[]  NOutMin=[]  NOutMax=[]  SumOutMin=[]  SumOutMax=[]  SaturationOutMin=[]  SaturationOutMax=[]  PParamMin=[]  PParamMax=[]  IParamMin=[]  IParamMax=[]  DParamMin=[]  DParamMax=[]  NParamMin=[]  NParamMax=[]  KbParamMin=[]  KbParamMax=[]  KtParamMin=[]  KtParamMax=[]  KbOutMin=[]  KbOutMax=[]  KtOutMin=[]  KtOutMax=[]  IntegratorOutMin=[]  IntegratorOutMax=[]  FilterOutMin=[]  FilterOutMax=[]  SumI1OutMin=[]  SumI1OutMax=[]  SumI2OutMin=[]  SumI2OutMax=[]  SumI3OutMin=[]  SumI3OutMax=[]  SumI4OutMin=[]  SumI4OutMax=[]  SumDOutMin=[]  SumDOutMax=[]  DifferentiatorOutMin=[]  DifferentiatorOutMax=[]  FilterDiffOutCoefMin=[]  FilterDiffOutCoefMax=[]  ReciprocalOutMin=[]  ReciprocalOutMax=[]  SumDenOutMin=[]  SumDenOutMax=[]  SumNumOutMin=[]  SumNumOutMax=[]  DivideOutMin=[]  DivideOutMax=[]  UdiffTsProdOutMin=[]  UdiffTsProdOutMax=[]  NTsProdOutMin=[]  NTsProdOutMax=[]  UintegralTsProdOutMin=[]  UintegralTsProdOutMax=[]  UngainTsProdOutMin=[]  UngainTsProdOutMax=[]  IntegratorContinuousStateAttributes=''  IntegratorStateMustResolveToSignalObject=off  IntegratorRTWStateStorageClass=Auto  FilterContinuousStateAttributes=''  FilterStateMustResolveToSignalObject=off  FilterRTWStateStorageClass=Auto  ParallelPVariant=InternalParameters  IdealPVariant=Disabled  IVariant=InternalParameters  DVariant=InternalParameters  IntegratorVariant=Discrete  SatVariant=Disabled  AWVariant=Passthrough  PCopyVariant=Disabled  TRVariant=Disabled  FdbkBlocksVariant=Forward  IdealPFdbkVariant=Disabled  SatFdbkVariant=Disabled  DerivativeFilterVariant=ForwardEulerFilter  NVariant=InternalParameters  NCopyVariant=Disabled  FilterICVariant=InternalICsFilter  IntegratorICVariant=InternalICs  ExternalResetVariant=Disabled  TRSumVariant=Passthrough  SumFdbkVariant=Disabled  SumVariant=Sum_PID  TsampFilterVariant=InternalTs  TsampNgainVariant=Passthrough  TsampIntegralVariant=Passthrough  ExternalSaturationOutDataTypeStr=Inherit: Same as second input
  Product : Product
  Product1 : Product
  Quaternions to Rotation Angles : sharedtransform/Quaternions to Rotation Angles  Commented=on  rotationOrder=XYZ  aMode=aMode
      settings: SourceProductBaseCode=AE,PW,DR,MT,UV,VE
  Sum : Sum  Inputs=+++
  Control torque [body frame] : Outport
  wires:
  Mux/1 -> Product/2
  Demux/1 -> Product/1
  Quaternions to Rotation Angles/1 -> Demux1/1
  Demux1/1 -> PID Controller/1
  Demux1/2 -> PID Controller1/1
  Demux1/3 -> PID Controller2/1
  PID Controller/1 -> Mux1/1
  PID Controller1/1 -> Mux1/2
  PID Controller2/1 -> Mux1/3
  OmegaErr [body frame]/1 -> Gain/1
  Sum/1 -> Control torque [body frame]/1
  AttitudeErr [body frame]/1 -> Demux/1
  Demux/2 -> Mux/1
  Demux/3 -> Mux/2
  Demux/4 -> Mux/3
  Product/1 -> Gain1/1
  Angular speed [body frame]/1 -> Product1/1, Cross Product/1
  Inertia/1 -> Product1/2
  Product1/1 -> Cross Product/2
  Cross Product/1 -> Sum/1
  Gain/1 -> Sum/2
  Gain1/1 -> Sum/3

== system main/QUEST/Angles 2 vector ==
  In1 : Inport
  Constant : Constant
  Demux : Demux  Outputs=2
  Demux1 : Demux  Outputs=3
  Divide : Product  Inputs=/*
  Mux : Mux  Inputs=3
  Sqrt : Sqrt  SaturateOnIntegerOverflow=on
  Square : Math  Operator=square  SaturateOnIntegerOverflow=on
  Sum : Sum  Inputs=+++
  Tan : Trigonometry  Operator=tan
  Out1 : Outport
  wires:
  Divide/1 -> Out1/1
  Square/1 -> Demux1/1
  Demux1/3 -> Sum/3
  Sum/1 -> Sqrt/1
  Demux/2 -> Mux/2
  Mux/1 -> Divide/2, Square/1
  Demux1/2 -> Sum/2
  In1/1 -> Tan/1
  Demux/1 -> Mux/1
  Sqrt/1 -> Divide/1
  Constant/1 -> Mux/3
  Tan/1 -> Demux/1
  Demux1/1 -> Sum/1

== system main/QUEST/Angles 2 vector1 ==
  Star 2 : Inport
  Constant : Constant
  Demux : Demux  Outputs=2
  Demux1 : Demux  Outputs=3
  Divide : Product  Inputs=/*
  Mux : Mux  Inputs=3
  Sqrt : Sqrt  SaturateOnIntegerOverflow=on
  Square : Math  Operator=square  SaturateOnIntegerOverflow=on
  Sum : Sum  Inputs=+++
  Tan : Trigonometry  Operator=tan
  Out1 : Outport
  wires:
  Divide/1 -> Out1/1
  Square/1 -> Demux1/1
  Demux1/3 -> Sum/3
  Sum/1 -> Sqrt/1
  Demux/2 -> Mux/2
  Mux/1 -> Divide/2, Square/1
  Demux1/2 -> Sum/2
  Star 2/1 -> Tan/1
  Demux/1 -> Mux/1
  Sqrt/1 -> Divide/1
  Constant/1 -> Mux/3
  Tan/1 -> Demux/1
  Demux1/1 -> Sum/1

== system main/QUEST/Angles 2 vector2 ==
  Star 3 : Inport
  Constant : Constant
  Demux : Demux  Outputs=2
  Demux1 : Demux  Outputs=3
  Divide : Product  Inputs=/*
  Mux : Mux  Inputs=3
  Sqrt : Sqrt  SaturateOnIntegerOverflow=on
  Square : Math  Operator=square  SaturateOnIntegerOverflow=on
  Sum : Sum  Inputs=+++
  Tan : Trigonometry  Operator=tan
  Out1 : Outport
  wires:
  Divide/1 -> Out1/1
  Square/1 -> Demux1/1
  Demux1/3 -> Sum/3
  Sum/1 -> Sqrt/1
  Demux/2 -> Mux/2
  Mux/1 -> Divide/2, Square/1
  Demux1/2 -> Sum/2
  Star 3/1 -> Tan/1
  Demux/1 -> Mux/1
  Sqrt/1 -> Divide/1
  Constant/1 -> Mux/3
  Tan/1 -> Demux/1
  Demux1/1 -> Sum/1

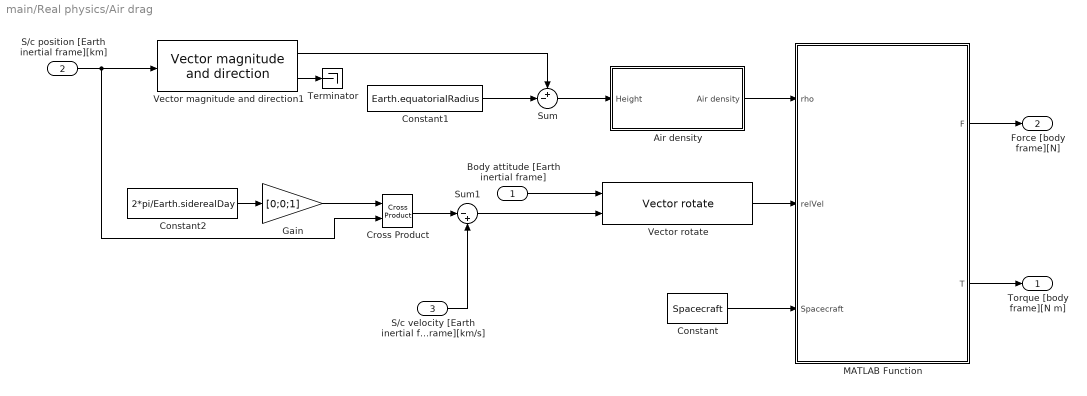
== system main/Real physics/Air drag ==
  Body attitude [Earth inertial frame] : Inport  Unit=1
  S/c position [Earth inertial frame][km] : Inport  Port=2  OutDataTypeStr=double  Unit=km  PortDimensions=3
  S/c velocity [Earth inertial frame][km/s] : Inport  Port=3  OutDataTypeStr=double  Unit=km/s
  Air density : Subsystem
  Constant : Constant  Value=Spacecraft  OutDataTypeStr=Bus: SpacecraftDT
  Constant1 : Constant  Value=Earth.equatorialRadius
  Constant2 : Constant  Value=2*pi/Earth.siderealDay
  Cross Product : vrlib/Utilities/Cross Product
  Gain : Gain  Gain=[0;0;1]
  MATLAB Function : MATLAB Function  TreatAsAtomicUnit=on
  Sum : Sum  Inputs=+-|
  Sum1 : Sum  Inputs=|-+
  Terminator : Terminator
  Vector magnitude and direction1 : SADlibrary/Vector magnitude and direction  SystemSampleTime=-1  VariantActivationTime=update diagram  Latency=0  AutoFrameSizeCalculation=off
  Vector rotate : SADlibrary/Vector rotate  SystemSampleTime=-1  VariantActivationTime=update diagram  Latency=0  AutoFrameSizeCalculation=off
  Torque [body frame][N m] : Outport  Unit=N*m
  Force [body frame][N] : Outport  Port=2  Unit=N
  wires:
  Vector magnitude and direction1/1 -> Sum/1
  Body attitude [Earth inertial frame]/1 -> Vector rotate/1
  MATLAB Function/2(T) -> Torque [body frame][N m]/1
  MATLAB Function/1(F) -> Force [body frame][N]/1
  Constant/1 -> MATLAB Function/3(Spacecraft)
  Vector rotate/1 -> MATLAB Function/2(relVel)
  Constant1/1 -> Sum/2
  Constant2/1 -> Gain/1
  Gain/1 -> Cross Product/1
  Cross Product/1 -> Sum1/1
  S/c velocity [Earth inertial frame][km/s]/1 -> Sum1/2
  Sum1/1 -> Vector rotate/2
  Sum/1 -> Air density/1(Height)
  Air density/1(Air density) -> MATLAB Function/1(rho)
  S/c position [Earth inertial frame][km]/1 -> Vector magnitude and direction1/1, Cross Product/2
  Vector magnitude and direction1/2 -> Terminator/1

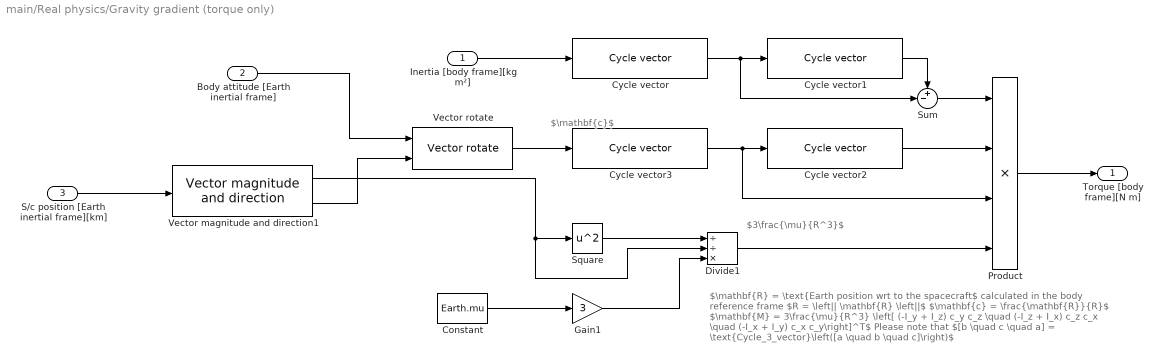
== system main/Real physics/Gravity gradient (torque only) ==
  note: $3\frac{\mu}{R^3}$
  note: $\mathbf{c}$
  note: $\mathbf{R} = \text{Earth position wrt to the spacecraft$ calculated in the body reference frame
      | $R = \left|| \mathbf{R} \left||$
      | $\mathbf{c} = \frac{\mathbf{R}}{R}$
      | $\mathbf{M} = 3\frac{\mu}{R^3} \left[ (-I_y + I_z) c_y c_z \quad (-I_z + I_x) c_z c_x \quad (-I_x + I_y) c_x c_y\right]^T$
      |
      | Please note that
      | $[b \quad c \quad a] = \text{Cycle_3_vector}\left([a \quad b \quad c]\right)$
  Inertia [body frame][kg m²] : Inport  Unit=kg*m^2
  Body attitude [Earth inertial frame] : Inport  Port=2  Unit=1
  S/c position [Earth inertial frame][km] : Inport  Port=3  OutDataTypeStr=double  Unit=km
  Constant : Constant  Value=Earth.mu
  Cycle vector{,1..3} (4 alike) : SADlibrary/Cycle vector  SystemSampleTime=-1  VariantActivationTime=update diagram  Latency=0  AutoFrameSizeCalculation=off
  Divide1 : Product  Inputs=//*
  Gain1 : Gain  Gain=3
  Product : Product  Inputs=4
  Square : Math  Operator=square  SaturateOnIntegerOverflow=on
  Sum : Sum  Inputs=+-|
  Vector magnitude and direction1 : SADlibrary/Vector magnitude and direction  SystemSampleTime=-1  VariantActivationTime=update diagram  Latency=0  AutoFrameSizeCalculation=off
  Vector rotate : SADlibrary/Vector rotate  SystemSampleTime=-1  VariantActivationTime=update diagram  Latency=0  AutoFrameSizeCalculation=off
  Torque [body frame][N m] : Outport  Unit=N*m
  wires:
  Inertia [body frame][kg m²]/1 -> Cycle vector/1
  Product/1 -> Torque [body frame][N m]/1
  Constant/1 -> Gain1/1
  Divide1/1 -> Product/4
  Cycle vector3/1 -> Product/3, Cycle vector2/1
  Cycle vector/1 -> Sum/2, Cycle vector1/1
  Cycle vector2/1 -> Product/2
  Cycle vector1/1 -> Sum/1
  Sum/1 -> Product/1
  Gain1/1 -> Divide1/3
  Square/1 -> Divide1/1
  Vector magnitude and direction1/1 -> Divide1/2, Square/1
  S/c position [Earth inertial frame][km]/1 -> Vector magnitude and direction1/1
  Vector magnitude and direction1/2 -> Vector rotate/2
  Vector rotate/1 -> Cycle vector3/1
  Body attitude [Earth inertial frame]/1 -> Vector rotate/1

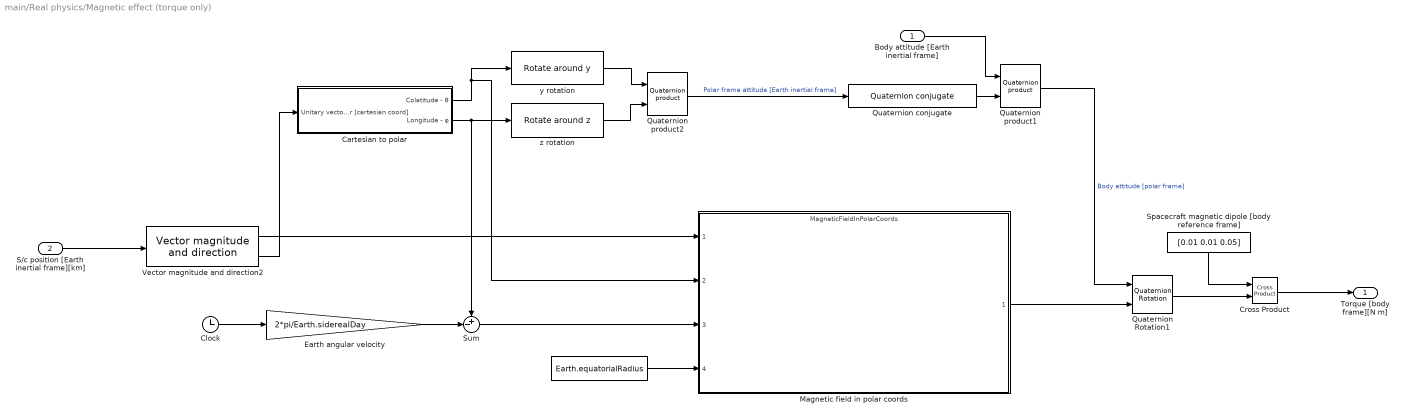
== system main/Real physics/Magnetic effect (torque only) ==
  Body attitude [Earth inertial frame] : Inport  Unit=1
  S/c position [Earth inertial frame][km] : Inport  Port=2  OutDataTypeStr=double  Unit=km
  " " : Constant  Value=Earth.equatorialRadius
  Cartesian to polar : Subsystem
  Clock : Clock
  Cross Product : vrlib/Utilities/Cross Product
  Earth angular velocity : Gain  Gain=2*pi/Earth.siderealDay
  Magnetic field in polar coords : ModelReference  ModelNameDialog=MagneticFieldInPolarCoords.slx  SimulationMode=Normal  ModelReferenceVersion=1.3
  Quaternion Rotation1 : aerolibutil/Quaternion Rotation
  Quaternion conjugate : SADlibrary/Quaternion conjugate  SystemSampleTime=-1  VariantActivationTime=update diagram  Latency=0  AutoFrameSizeCalculation=off
  Quaternion product1 : SADlibrary/Quaternion product  SystemSampleTime=-1  VariantActivationTime=update diagram  Latency=0  AutoFrameSizeCalculation=off
  Quaternion product2 : SADlibrary/Quaternion product  SystemSampleTime=-1  VariantActivationTime=update diagram  Latency=0  AutoFrameSizeCalculation=off
  Spacecraft magnetic dipole [body reference frame] : Constant  Value=[0.01 0.01 0.05]
  Sum : Sum  Inputs=+-|
  Vector magnitude and direction2 : SADlibrary/Vector magnitude and direction  SystemSampleTime=-1  VariantActivationTime=update diagram  Latency=0  AutoFrameSizeCalculation=off
  y rotation : SADlibrary/Rotate around y  SystemSampleTime=-1  VariantActivationTime=update diagram  Latency=0  AutoFrameSizeCalculation=off
  z rotation : SADlibrary/Rotate around z  SystemSampleTime=-1  VariantActivationTime=update diagram  Latency=0  AutoFrameSizeCalculation=off
  Torque [body frame][N m] : Outport  OutDataTypeStr=double  Unit=N*m
  wires:
  Cartesian to polar/2(Longitude - φ) -> z rotation/1, Sum/1
  Cartesian to polar/1(Colatitude - θ) -> y rotation/1, Magnetic field in polar coords/2
  y rotation/1 -> Quaternion product2/1
  z rotation/1 -> Quaternion product2/2
  Quaternion product2/1 -> Quaternion conjugate/1  "Polar frame attitude [Earth inertial frame]"
  Body attitude [Earth inertial frame]/1 -> Quaternion product1/1
  Quaternion conjugate/1 -> Quaternion product1/2
  Quaternion product1/1 -> Quaternion Rotation1/1  "Body attitude [polar frame]"
  Clock/1 -> Earth angular velocity/1
  Earth angular velocity/1 -> Sum/2
  Sum/1 -> Magnetic field in polar coords/3
  " "/1 -> Magnetic field in polar coords/4
  Spacecraft magnetic dipole [body reference frame]/1 -> Cross Product/1
  Quaternion Rotation1/1 -> Cross Product/2
  Cross Product/1 -> Torque [body frame][N m]/1
  Magnetic field in polar coords/1 -> Quaternion Rotation1/2
  Vector magnitude and direction2/2 -> Cartesian to polar/1(Unitary vector [cartesian coord])
  Vector magnitude and direction2/1 -> Magnetic field in polar coords/1
  S/c position [Earth inertial frame][km]/1 -> Vector magnitude and direction2/1
